simulink library "lib_Radiation_HeatXCoeffNonRefSink"  (R2015a)
settings: Solver=ode45  StartTime=0.0  StopTime=10.0  RelTol=1e-3
settings Model: Creator=jlkratz  LastModifiedBy=jlkratz

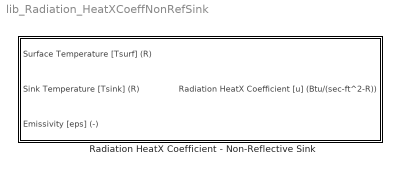
== system lib_Radiation_HeatXCoeffNonRefSink ==
  Radiation HeatX Coefficient - Non-Reflective Sink : Subsystem  mask(TSAT: Radiation HeatX Coefficient - Non-Reflective Sink Block){}
      mask help:
      | This function computes the radiation heat transfer coefficient when the radiation term is written in a linear form (q = u*(Text - Tsurf)). This block is applicable for radiation between a surface and a non-reflective sink such as a distant black body.
      |
      | Units are specified on the inport and outports so be sure to adhere to the appropriate units.
      mask Help: web(which('Radiation_TSAT_HeatXCoeffNonRefSink.html'),'-helpbrowser')

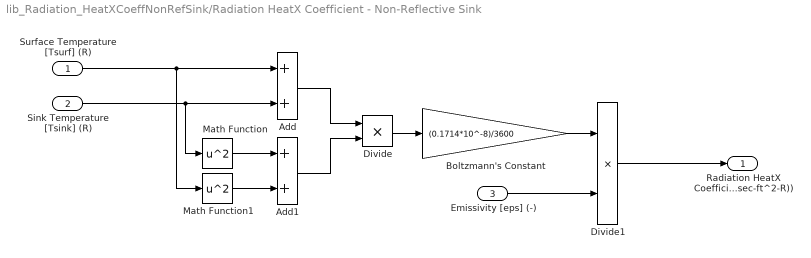
== system lib_Radiation_HeatXCoeffNonRefSink/Radiation HeatX Coefficient - Non-Reflective Sink ==
  Surface Temperature [Tsurf] (R) : Inport
  Sink Temperature [Tsink] (R) : Inport  Port=2
  Emissivity [eps] (-) : Inport  Port=3
  Add : Sum
  Add1 : Sum
  Boltzmann's Constant : Gain  Gain=(0.1714*10^-8)/3600
  Divide : Product  Inputs=**
  Divide1 : Product  Inputs=**
  Math Function : Math  Operator=square  SaturateOnIntegerOverflow=on
  Math Function1 : Math  Operator=square  SaturateOnIntegerOverflow=on
  Radiation HeatX Coefficient [u] (Btu/(sec-ft^2-R)) : Outport
  wires:
  Math Function1/1 -> Add1/2
  Divide1/1 -> Radiation HeatX Coefficient [u] (Btu/(sec-ft^2-R))/1
  Surface Temperature [Tsurf] (R)/1 -> Add/1, Math Function1/1
  Sink Temperature [Tsink] (R)/1 -> Add/2, Math Function/1
  Divide/1 -> Boltzmann's Constant/1
  Emissivity [eps] (-)/1 -> Divide1/2
  Add1/1 -> Divide/2
  Boltzmann's Constant/1 -> Divide1/1
  Add/1 -> Divide/1
  Math Function/1 -> Add1/1
